simulink library "models"  (Simulink 6.3)
undefined symbols (not defined in the file or in its folder): aero, airplane2body, body2airplane, bspan, cbar, constants, Sref, trac_params, vehicle_params
libraries: model_lib x5, models x3, simulink x2, utility_lib x1
settings Model: LastModifiedBy=E700252

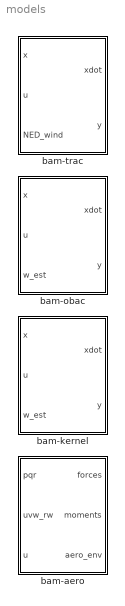
== system models ==
  bam-aero : Subsystem  mask{aero_params=aero}
      mask prompts: aero_params "aero params"
      mask init:
      | paramnames = fieldnames(aero_params);
      | for i=1:length(paramnames)
      | 	eval([paramnames{i} '= aero_params.' paramnames{i} ';']);
      | end
  bam-kernel : Subsystem  mask{vehicle_params=vehicle_params}
      mask prompts: vehicle_params "vehicle params"
      mask init:
      | paramnames = fieldnames(vehicle_params);
      | for i=1:length(paramnames)
      | 	eval([paramnames{i} '= vehicle_params.' paramnames{i} ';']);
      | end
  bam-obac : Subsystem
  bam-trac : Subsystem  mask{vehicle_params=trac_params}
      mask prompts: vehicle_params "vehicle params"

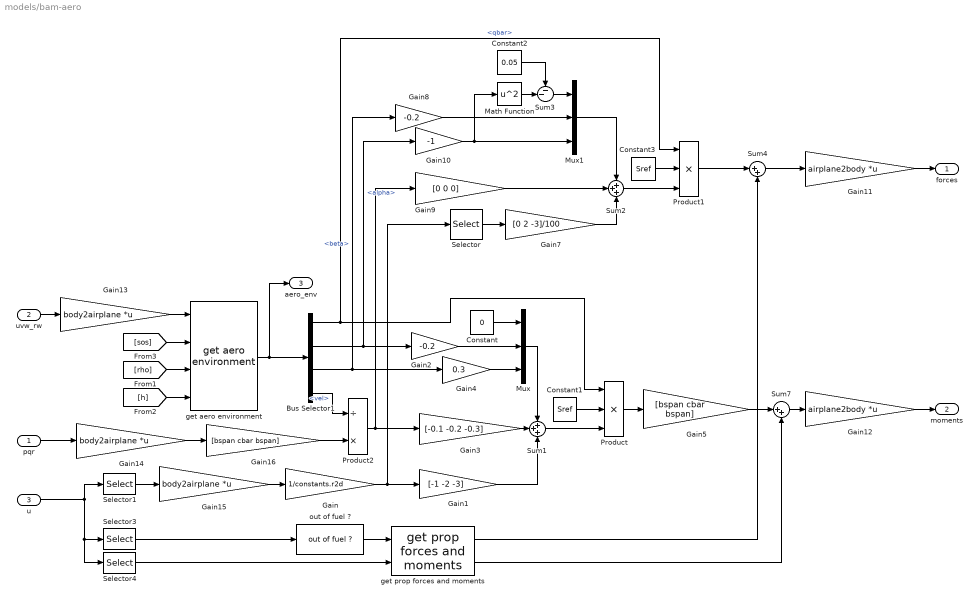
== system models/bam-aero ==
  pqr : Inport
  uvw_rw : Inport  Port=2
  u : Inport  Port=3
  Bus Selector1 : BusSelector  OutputSignals=qbar,alpha,beta,vel
  Constant : Constant  Value=0
  Constant1 : Constant  Value=Sref
  Constant2 : Constant  Value=0.05
  Constant3 : Constant  Value=Sref
  Gain : Gain  Gain=1/constants.r2d
  Gain1 : Gain  Gain=[-1 -2 -3]
  Gain10 : Gain  Gain=-1
  Gain11 : Gain  Gain=airplane2body  Multiplication=Matrix(K*u)
  Gain12 : Gain  Gain=airplane2body  Multiplication=Matrix(K*u)
  Gain13 : Gain  Gain=body2airplane  Multiplication=Matrix(K*u)
  Gain14 : Gain  Gain=body2airplane  Multiplication=Matrix(K*u)
  Gain15 : Gain  Gain=body2airplane  Multiplication=Matrix(K*u)
  Gain16 : Gain  Gain=[bspan cbar bspan]
  Gain2 : Gain  Gain=-0.2
  Gain3 : Gain  Gain=[-0.1 -0.2 -0.3]
  Gain4 : Gain  Gain=0.3
  Gain5 : Gain  Gain=[bspan cbar bspan]
  Gain7 : Gain  Gain=[0 2 -3]/100
  Gain8 : Gain  Gain=-0.2
  Gain9 : Gain  Gain=[0 0 0]
  Math Function : Math  Operator=square  SaturateOnIntegerOverflow=on
  Mux : Mux  Inputs=3
  Mux1 : Mux  Inputs=3
  Product : Product  Inputs=3  RndMeth=Zero
  Product1 : Product  Inputs=3  RndMeth=Zero
  Product2 : Product  Inputs=/*  RndMeth=Zero
  Selector : Selector  Elements=[1 3 2]  InputPortWidth=3
  Selector1 : Selector  Elements=vane_idx  InputPortWidth=num_u
  Selector3 : Selector  Elements=throttle_idx  InputPortWidth=num_u
  Selector4 : Selector  Elements=tvc_idx  InputPortWidth=num_u
  Sum1 : Sum  Inputs=+++
  Sum2 : Sum  Inputs=+++
  Sum3 : Sum  Inputs=--|
  Sum4 : Sum  Inputs=|++
  Sum7 : Sum  Inputs=|++
  get aero environment : model_lib/get aero environment
  get prop forces and moments : model_lib/get prop forces and moments
  out of fuel ? : model_lib/out of fuel ?
  forces : Outport
  moments : Outport  Port=2
  aero_env : Outport  Port=3
  wires:
  Selector/1 -> Gain7/1
  get prop forces and moments/1 -> Sum4/2
  out of fuel ?/1 -> get prop forces and moments/1
  Selector4/1 -> get prop forces and moments/2
  Selector3/1 -> out of fuel ?/1
  get prop forces and moments/2 -> Sum7/2
  Gain5/1 -> Sum7/1
  Sum7/1 -> Gain12/1
  get aero environment/1 -> aero_env/1, Bus Selector1/1
  [h] -> get aero environment/4
  [sos] -> get aero environment/2
  Gain13/1 -> get aero environment/1
  [rho] -> get aero environment/3
  Selector1/1 -> Gain15/1
  Bus Selector1/4 -> Product2/1  "<vel>"
  Product2/1 -> Gain9/1, Gain3/1
  Gain16/1 -> Product2/2
  Gain15/1 -> Gain/1
  Sum4/1 -> Gain11/1
  Product1/1 -> Sum4/1
  Gain14/1 -> Gain16/1
  Gain12/1 -> moments/1
  Gain11/1 -> forces/1
  Sum3/1 -> Mux1/1
  Math Function/1 -> Sum3/2
  Constant2/1 -> Sum3/1
  Constant3/1 -> Product1/2
  Sum2/1 -> Product1/3
  Gain7/1 -> Sum2/3
  Gain9/1 -> Sum2/2
  Mux1/1 -> Sum2/1
  Gain8/1 -> Mux1/2
  Gain10/1 -> Math Function/1, Mux1/3
  Product/1 -> Gain5/1
  Constant1/1 -> Product/2
  Bus Selector1/1 -> Product/1, Product1/1  "<qbar>"
  Sum1/1 -> Product/3
  Gain1/1 -> Sum1/3
  Gain3/1 -> Sum1/2
  Mux/1 -> Sum1/1
  Constant/1 -> Mux/1
  Gain2/1 -> Mux/2
  Gain4/1 -> Mux/3
  Bus Selector1/3 -> Gain8/1, Gain4/1  "<beta>"
  pqr/1 -> Gain14/1
  Bus Selector1/2 -> Gain10/1, Gain2/1  "<alpha>"
  Gain/1 -> Selector/1, Gain1/1
  u/1 -> Selector4/1, Selector3/1, Selector1/1
  uvw_rw/1 -> Gain13/1

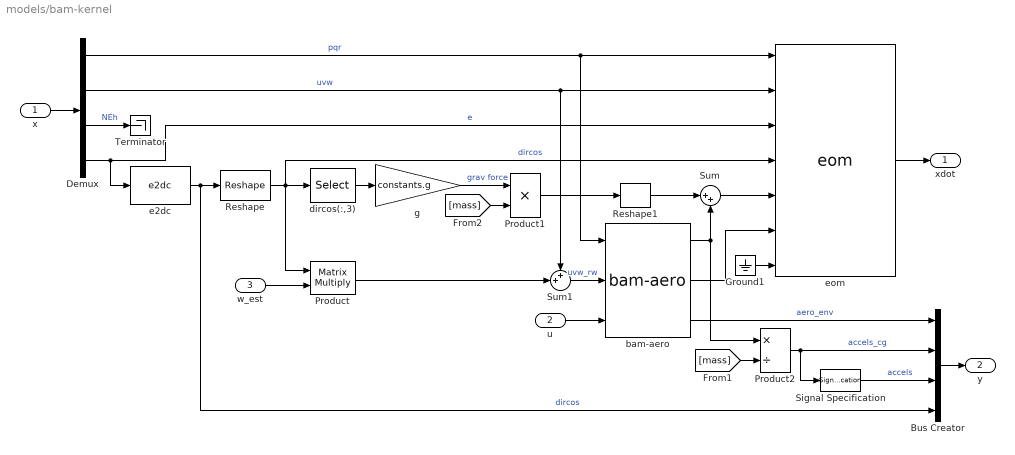
== system models/bam-kernel ==
  x : Inport
  u : Inport  Port=2
  w_est : Inport  Port=3
  Bus Creator : BusCreator
  Demux : Demux  Outputs=[3 3 3 4]
  Ground1 : Ground
  Product : Product  Multiplication=Matrix(*)  SaturateOnIntegerOverflow=on
  Product1 : Product  RndMeth=Zero
  Product2 : Product  Inputs=*/  RndMeth=Zero
  Reshape : simulink/Math Operations/Reshape  OutputDimensionality=Customize  OutputDimensions=[3,3]
  Reshape1 : simulink/Math Operations/Reshape  OutputDimensionality=1-D array  OutputDimensions=[1,1]
  Signal Specification : SignalSpecification  Dimensions=3
  Sum : Sum  Inputs=|++  SaturateOnIntegerOverflow=on
  Sum1 : Sum  Inputs=++|  SaturateOnIntegerOverflow=on
  Terminator : Terminator
  bam-aero : models/bam-aero  aero_params=aero
  dircos(:,3) : Selector  InputType=Matrix  Elements=[7:9]  Rows=-1  Columns=3  InputPortWidth=9
  e2dc : utility_lib/e2dc
  eom : model_lib/eom
  g : Gain  Gain=constants.g  SaturateOnIntegerOverflow=on
  xdot : Outport
  y : Outport  Port=2
  wires:
  Ground1/1 -> eom/7
  Product1/1 -> Reshape1/1
  [mass] -> Product1/2
  g/1 -> Product1/1  "grav force"
  x/1 -> Demux/1
  Demux/1 -> eom/1, bam-aero/1  "pqr"
  Demux/3 -> Terminator/1  "NEh"
  Demux/4 -> eom/3, e2dc/1  "e"
  Demux/2 -> eom/2, Sum1/1  "uvw"
  dircos(:,3)/1 -> g/1
  eom/1 -> xdot/1
  e2dc/1 -> Reshape/1, Bus Creator/4  "dircos"
  u/1 -> bam-aero/3
  bam-aero/1 -> Sum/2, Product2/1
  Sum1/1 -> bam-aero/2  "uvw_rw"
  w_est/1 -> Product/2
  Product/1 -> Sum1/2
  Sum/1 -> eom/5
  Reshape/1 -> eom/4, dircos(:,3)/1, Product/1  "dircos"
  bam-aero/2 -> eom/6
  bam-aero/3 -> Bus Creator/1  "aero_env"
  Product2/1 -> Bus Creator/2, Signal Specification/1  "accels_cg"
  [mass] -> Product2/2
  Signal Specification/1 -> Bus Creator/3  "accels"
  Bus Creator/1 -> y/1
  Reshape1/1 -> Sum/1

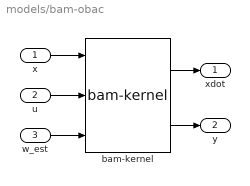
== system models/bam-obac ==
  x : Inport
  u : Inport  Port=2
  w_est : Inport  Port=3
  bam-kernel : models/bam-kernel  vehicle_params=obac_params
  xdot : Outport
  y : Outport  Port=2
  wires:
  bam-kernel/2 -> y/1
  bam-kernel/1 -> xdot/1
  w_est/1 -> bam-kernel/3
  u/1 -> bam-kernel/2
  x/1 -> bam-kernel/1

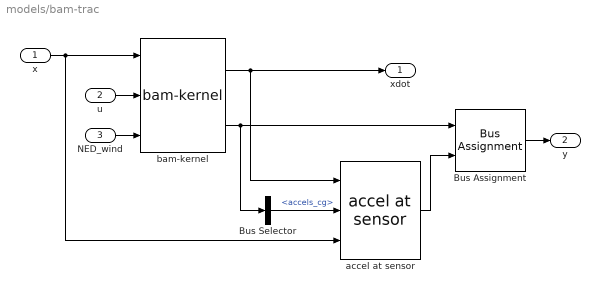
== system models/bam-trac ==
  x : Inport
  u : Inport  Port=2
  NED_wind : Inport  Port=3
  Bus Assignment : BusAssignment  AssignedSignals=accels
  Bus Selector : BusSelector  OutputSignals=accels_cg
  accel at sensor : model_lib/accel at sensor  vehicle_params=vehicle_params
  bam-kernel : models/bam-kernel  vehicle_params=vehicle_params
  xdot : Outport
  y : Outport  Port=2
  wires:
  Bus Assignment/1 -> y/1
  NED_wind/1 -> bam-kernel/3
  x/1 -> bam-kernel/1, accel at sensor/3
  u/1 -> bam-kernel/2
  bam-kernel/1 -> xdot/1, accel at sensor/1
  accel at sensor/1 -> Bus Assignment/2
  bam-kernel/2 -> Bus Selector/1, Bus Assignment/1
  Bus Selector/1 -> accel at sensor/2  "<accels_cg>"
